simulink model "Lab6_task1"  (R2021b)
settings: Solver=VariableStepAuto  StartTime=0.0  StopTime=10.0  RelTol=1e-3
values from neighbouring files (symbols this model uses):
  A0 = eye(3)    [Lab08_script.m]    (also in Lab7_script.m; Lab7_scriptscalar.m; Lab_GG.m)
  I = [Ix 0 0; 0 Iy 0; 0 0 Iz]    [Lab08_script.m]    (also in Lab7_script.m; Lab7_scriptscalar.m; Lab_GG.m)
  I_inv = inv(I)    [Lab08_script.m]    (also in Lab7_script.m; Lab7_scriptscalar.m; Lab_GG.m)
  n = 10    [Chapter3.m]    (also in Lab08_script.m = sqrt(mu_E/(a^3)); Lab7_script.m = sqrt(mu_E/(a^3)); Lab7_scriptscalar.m = sqrt(mu_E/(a^3)); Lab_GG.m = sqrt(mu_E/(R_E+ r_orbit)^3))
  v1 = [Y1(:,4) Y1(:,5) Y1(:,6)]    [Excercise2_2223.m]    (also in Lab08_script.m = [0 1 -1]'; Lab7_script.m = [0 1 -1]'; Lab7_scriptscalar.m = [0 1 -1]'; Lab_GG.m = [0 1 -1]')
  v2 = [Y2(:,4) Y2(:,5) Y2(:,6)]    [Excercise2_2223.m]    (also in Lab08_script.m = [-1 0 1]'; Lab7_script.m = [-1 0 1]'; Lab7_scriptscalar.m = [-1 0 1]'; Lab_GG.m = [-1 0 1]')
  v3 = [1 -1 0]'    [Lab08_script.m]    (also in Lab7_script.m; Lab7_scriptscalar.m; Lab_GG.m)
  w_0 = [wx_0 wy_0 wz_0]'    [Lab08_script.m]    (also in Lab7_script.m; Lab7_scriptscalar.m; Lab_GG.m)
  w_L = [0 0 n]'    [Lab7_script.m]    (also in Lab7_scriptscalar.m; Lab_GG.m)
libraries: matrix_library x1
settings Model: Creator=sferl  LastModifiedBy=sferl

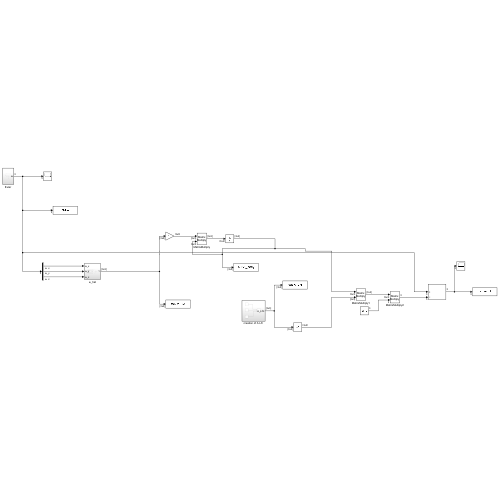
[thumbnail: Simulink's stored preview of the top-level diagram]
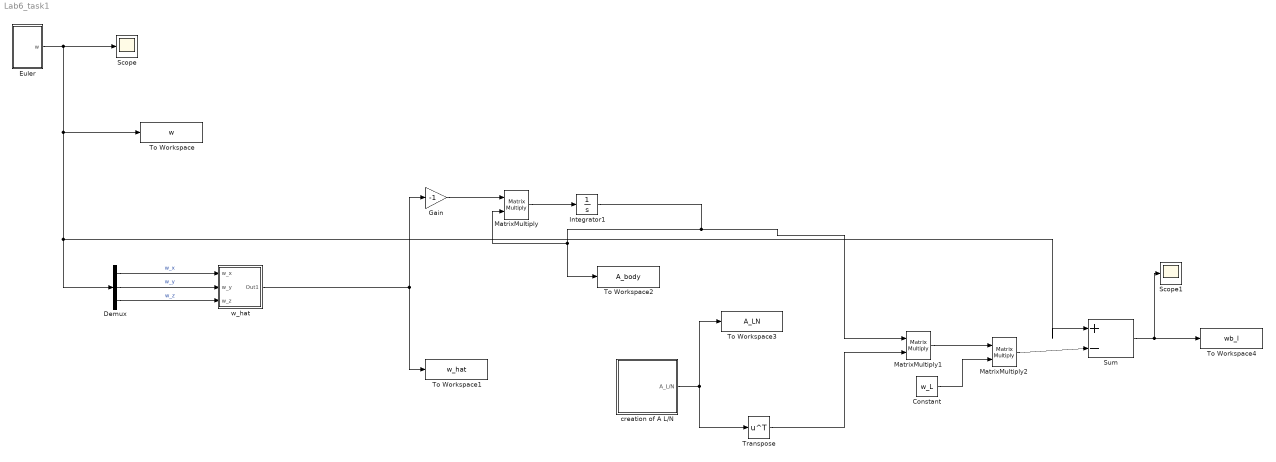
== system Lab6_task1 ==
  Constant : Constant  Value=w_L
  Demux : Demux  Outputs=3
  Euler : Subsystem
  Gain : Gain  Gain=-1
  Integrator1 : Integrator  InitialCondition=A0
  MatrixMultiply : Product  Multiplication=Matrix(*)
  MatrixMultiply1 : Product  Multiplication=Matrix(*)
  MatrixMultiply2 : Product  Multiplication=Matrix(*)
  Scope : Scope
  Scope1 : Scope
  Sum : Sum  Inputs=|+-
  To Workspace : ToWorkspace  VariableName=w  SampleTime=-1
  To Workspace1 : ToWorkspace  VariableName=w_hat  SampleTime=-1
  To Workspace2 : ToWorkspace  VariableName=A_body  SampleTime=-1
  To Workspace3 : ToWorkspace  VariableName=A_LN  SaveFormat=Timeseries  SampleTime=-1
  To Workspace4 : ToWorkspace  VariableName=wb_l  SampleTime=-1
  Transpose : Math  Operator=transpose  SaturateOnIntegerOverflow=on
  creation of A L/N : Subsystem
  w_hat : Subsystem
  wires:
  Gain/1 -> MatrixMultiply/1
  MatrixMultiply/1 -> Integrator1/1
  Integrator1/1 -> MatrixMultiply1/1, MatrixMultiply/2, To Workspace2/1
  Euler/1(w) -> Scope/1, Sum/1, Demux/1, To Workspace/1
  w_hat/1(Out1) -> Gain/1, To Workspace1/1
  Demux/1 -> w_hat/1(w_x)  "w_x"
  Demux/2 -> w_hat/2(w_y)  "w_y"
  Demux/3 -> w_hat/3(w_z)  "w_z"
  creation of A L/N/1(A_L/N) -> Transpose/1, To Workspace3/1
  Transpose/1 -> MatrixMultiply1/2
  MatrixMultiply1/1 -> MatrixMultiply2/1
  Constant/1 -> MatrixMultiply2/2
  MatrixMultiply2/1 -> Sum/2
  Sum/1 -> Scope1/1, To Workspace4/1

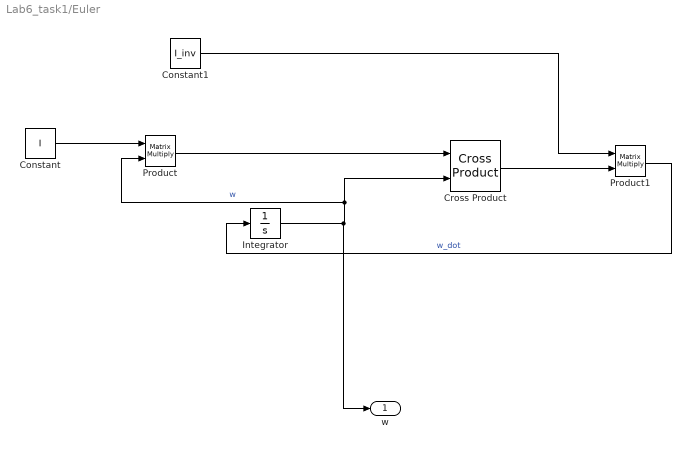
== system Lab6_task1/Euler ==
  Constant : Constant  Value=I  VectorParams1D=off
  Constant1 : Constant  Value=I_inv  VectorParams1D=off
  Cross Product : matrix_library/Cross Product
      settings: SourceProductBaseCode=SL
  Integrator : Integrator  InitialCondition=w_0
  Product : Product  Multiplication=Matrix(*)
  Product1 : Product  Multiplication=Matrix(*)
  w : Outport
  wires:
  Product/1 -> Cross Product/1
  Constant/1 -> Product/1
  Constant1/1 -> Product1/1
  Cross Product/1 -> Product1/2
  Integrator/1 -> w/1, Cross Product/2, Product/2  "w"
  Product1/1 -> Integrator/1  "w_dot"

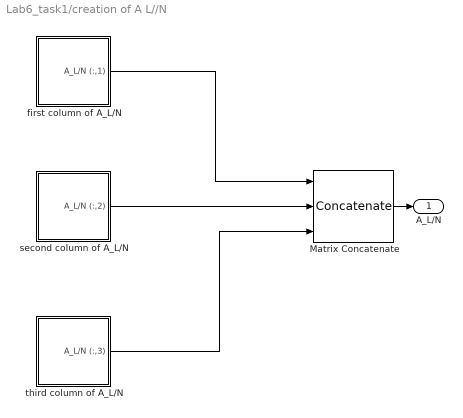
== system Lab6_task1/creation of A L//N ==
  Matrix Concatenate : Concatenate  NumInputs=3  Mode=Multidimensional array  ConcatenateDimension=2
  first column of A_L/N : Subsystem
  second column of A_L/N : Subsystem
  third column of A_L/N : Subsystem
  A_L/N : Outport
  wires:
  second column of A_L/N/1(A_L/N (:,2)) -> Matrix Concatenate/2
  Matrix Concatenate/1 -> A_L/N/1
  first column of A_L/N/1(A_L/N (:,1)) -> Matrix Concatenate/1
  third column of A_L/N/1(A_L/N (:,3)) -> Matrix Concatenate/3

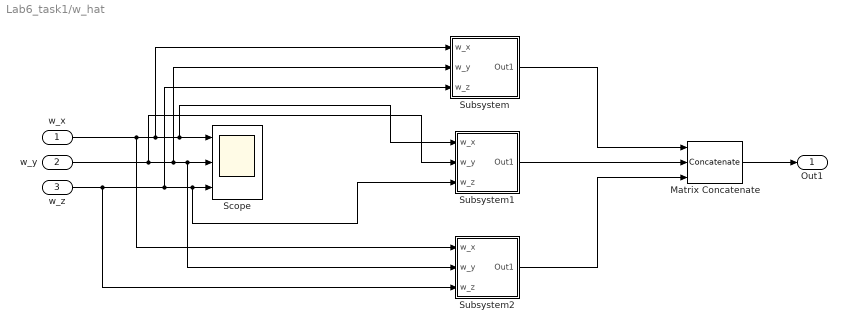
== system Lab6_task1/w_hat ==
  w_x : Inport
  w_y : Inport  Port=2
  w_z : Inport  Port=3
  Matrix Concatenate : Concatenate  NumInputs=3  Mode=Multidimensional array  ConcatenateDimension=2
  Scope : Scope  NumInputPorts=3
  Subsystem : Subsystem
  Subsystem1 : Subsystem
  Subsystem2 : Subsystem
  Out1 : Outport
  wires:
  w_y/1 -> Subsystem1/2(w_y), Subsystem/2(w_y), Subsystem2/2(w_y), Scope/2
  w_z/1 -> Subsystem2/3(w_z), Subsystem/3(w_z), Subsystem1/3(w_z), Scope/3
  w_x/1 -> Subsystem2/1(w_x), Subsystem/1(w_x), Subsystem1/1(w_x), Scope/1
  Subsystem2/1(Out1) -> Matrix Concatenate/3
  Subsystem1/1(Out1) -> Matrix Concatenate/2
  Subsystem/1(Out1) -> Matrix Concatenate/1
  Matrix Concatenate/1 -> Out1/1

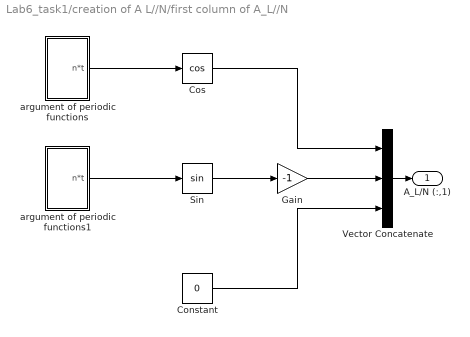
== system Lab6_task1/creation of A L//N/first column of A_L//N ==
  Constant : Constant  Value=0
  Cos : Trigonometry  Operator=cos
  Gain : Gain  Gain=-1
  Sin : Trigonometry
  Vector Concatenate : Concatenate  NumInputs=3
  argument of periodic functions : Subsystem
  argument of periodic functions1 : Subsystem
  A_L/N (:,1) : Outport
  wires:
  argument of periodic functions/1(n*t) -> Cos/1
  Constant/1 -> Vector Concatenate/3
  Cos/1 -> Vector Concatenate/1
  Vector Concatenate/1 -> A_L/N (:,1)/1
  Gain/1 -> Vector Concatenate/2
  Sin/1 -> Gain/1
  argument of periodic functions1/1(n*t) -> Sin/1

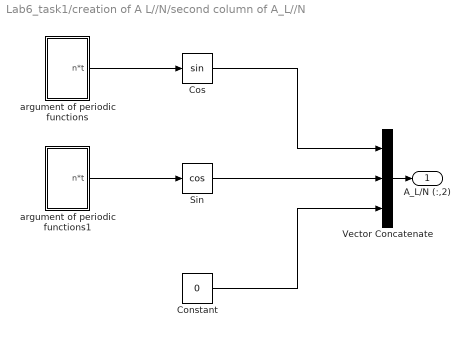
== system Lab6_task1/creation of A L//N/second column of A_L//N ==
  Constant : Constant  Value=0
  Cos : Trigonometry
  Sin : Trigonometry  Operator=cos
  Vector Concatenate : Concatenate  NumInputs=3
  argument of periodic functions : Subsystem
  argument of periodic functions1 : Subsystem
  A_L/N (:,2) : Outport
  wires:
  argument of periodic functions/1(n*t) -> Cos/1
  Constant/1 -> Vector Concatenate/3
  Cos/1 -> Vector Concatenate/1
  Vector Concatenate/1 -> A_L/N (:,2)/1
  Sin/1 -> Vector Concatenate/2
  argument of periodic functions1/1(n*t) -> Sin/1

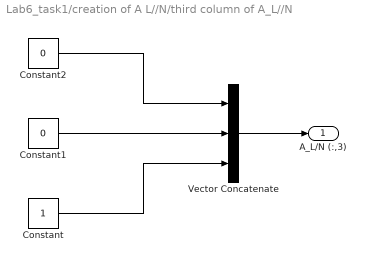
== system Lab6_task1/creation of A L//N/third column of A_L//N ==
  Constant : Constant
  Constant1 : Constant  Value=0
  Constant2 : Constant  Value=0
  Vector Concatenate : Concatenate  NumInputs=3
  A_L/N (:,3) : Outport
  wires:
  Constant/1 -> Vector Concatenate/3
  Vector Concatenate/1 -> A_L/N (:,3)/1
  Constant1/1 -> Vector Concatenate/2
  Constant2/1 -> Vector Concatenate/1

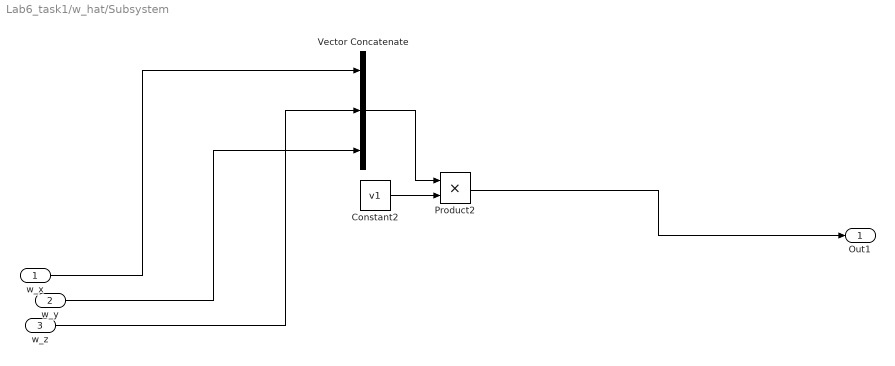
== system Lab6_task1/w_hat/Subsystem ==
  w_x : Inport
  w_y : Inport  Port=2
  w_z : Inport  Port=3
  Constant2 : Constant  Value=v1
  Product2 : Product
  Vector Concatenate : Concatenate  NumInputs=3
  Out1 : Outport
  wires:
  Product2/1 -> Out1/1
  Vector Concatenate/1 -> Product2/1
  Constant2/1 -> Product2/2
  w_x/1 -> Vector Concatenate/1
  w_z/1 -> Vector Concatenate/2
  w_y/1 -> Vector Concatenate/3

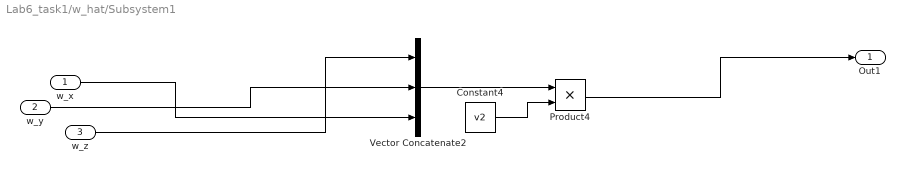
== system Lab6_task1/w_hat/Subsystem1 ==
  w_x : Inport
  w_y : Inport  Port=2
  w_z : Inport  Port=3
  Constant4 : Constant  Value=v2
  Product4 : Product
  Vector Concatenate2 : Concatenate  NumInputs=3
  Out1 : Outport
  wires:
  Constant4/1 -> Product4/2
  Vector Concatenate2/1 -> Product4/1
  Product4/1 -> Out1/1
  w_x/1 -> Vector Concatenate2/3
  w_y/1 -> Vector Concatenate2/2
  w_z/1 -> Vector Concatenate2/1

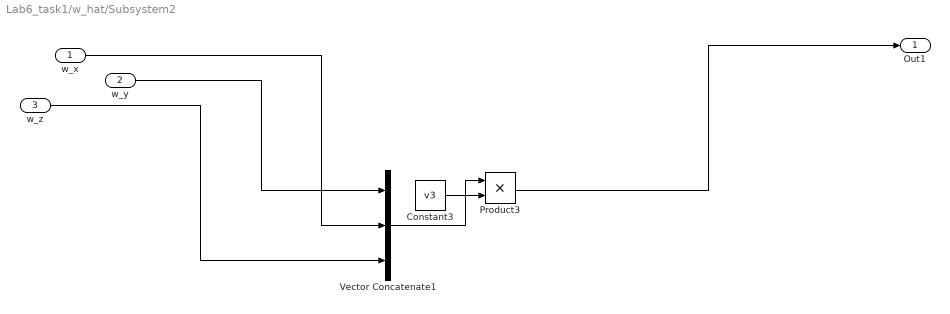
== system Lab6_task1/w_hat/Subsystem2 ==
  w_x : Inport
  w_y : Inport  Port=2
  w_z : Inport  Port=3
  Constant3 : Constant  Value=v3
  Product3 : Product
  Vector Concatenate1 : Concatenate  NumInputs=3
  Out1 : Outport
  wires:
  Product3/1 -> Out1/1
  Constant3/1 -> Product3/2
  w_y/1 -> Vector Concatenate1/1
  Vector Concatenate1/1 -> Product3/1
  w_x/1 -> Vector Concatenate1/2
  w_z/1 -> Vector Concatenate1/3

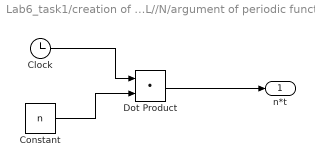
== system Lab6_task1/creation of A L//N/first column of A_L//N/argument of periodic functions ==
  Clock : Clock
  Constant : Constant  Value=n
  Dot Product : DotProduct  InputSameDT=on  OutDataTypeStr=Inherit: Inherit via internal rule
  n*t : Outport
  wires:
  Clock/1 -> Dot Product/1
  Dot Product/1 -> n*t/1
  Constant/1 -> Dot Product/2

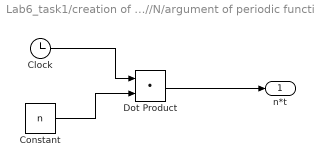
== system Lab6_task1/creation of A L//N/first column of A_L//N/argument of periodic functions1 ==
  Clock : Clock
  Constant : Constant  Value=n
  Dot Product : DotProduct  InputSameDT=on  OutDataTypeStr=Inherit: Inherit via internal rule
  n*t : Outport
  wires:
  Clock/1 -> Dot Product/1
  Dot Product/1 -> n*t/1
  Constant/1 -> Dot Product/2

== system Lab6_task1/creation of A L//N/second column of A_L//N/argument of periodic functions ==
  Clock : Clock
  Constant : Constant  Value=n
  Dot Product : DotProduct  InputSameDT=on  OutDataTypeStr=Inherit: Inherit via internal rule
  n*t : Outport
  wires:
  Clock/1 -> Dot Product/1
  Dot Product/1 -> n*t/1
  Constant/1 -> Dot Product/2

== system Lab6_task1/creation of A L//N/second column of A_L//N/argument of periodic functions1 ==
  Clock : Clock
  Constant : Constant  Value=n
  Dot Product : DotProduct  InputSameDT=on  OutDataTypeStr=Inherit: Inherit via internal rule
  n*t : Outport
  wires:
  Clock/1 -> Dot Product/1
  Dot Product/1 -> n*t/1
  Constant/1 -> Dot Product/2
